simulink model "CartesianSpace_Task"  (R2020b)
settings: Solver=FixedStepDiscrete  StartTime=0.0  StopTime=6  FixedStep=0.01  RelTol=1e-3
undefined symbols (not defined in the file): DiscIntNeverNeededParam
libraries: Utilities x6, robotcorelib x4, simulink x2, XBotBlockToolbox x2

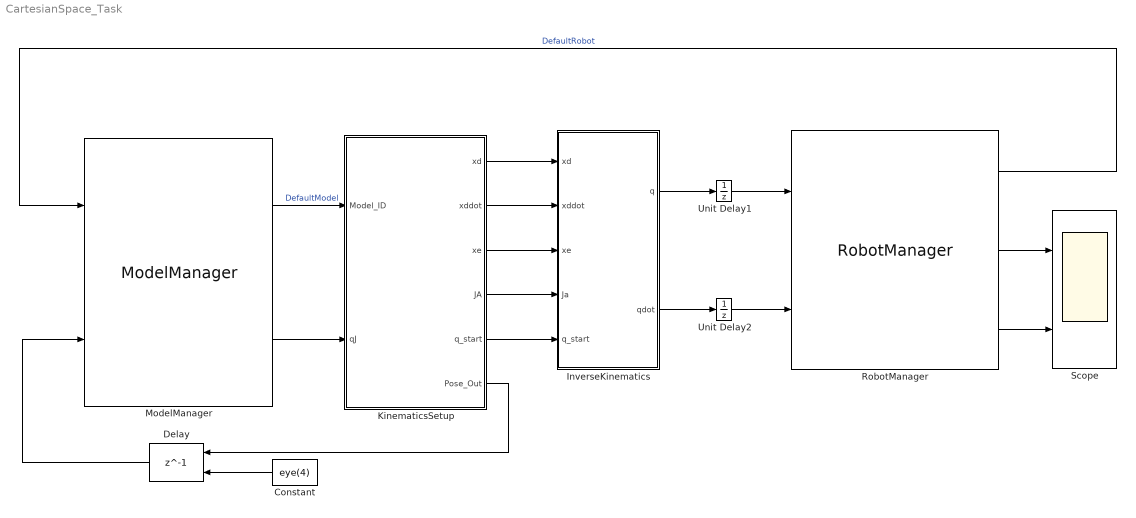
== system CartesianSpace_Task ==
  Constant : Constant  Value=eye(4)
  Delay : Delay  DelayLength=1  InitialConditionSource=Input port  InitialCondition=0
  InverseKinematics : Subsystem
  KinematicsSetup : Subsystem
  ModelManager : XBotBlockToolbox/ModelManager  ModelName=DefaultModel  RobotName=DefaultRobot  UseExtModel=Off  SyncWithRobot=On  GetFloatingBaseList={}  SetFloatingBaseComponent=Pose  GravityRequest=Off  ReadingsList={ 'qJ' }  MechanicalLimitsList={}  MechanicalLimitsCheck=Off  MechanicalLimitsEnforce=Off  SensorList={}  ReferencesList={}  OldModelName=DefaultModel
  RobotManager : XBotBlockToolbox/RobotManager  RobotName=DefaultRobot  ModelName=DefaultModel  UseExtRobot=Off  SyncWithModel=Off  ReadingsList={ 'qJ', 'qJdot' }  MechanicalLimitsList={}  MechanicalLimitsCheck=Off  MechanicalLimitsEnforce=Off  SensorList={}  ReferencesList={ 'qJ_ref', 'qJdot_ref' }  OldRobotName=DefaultRobot
  Scope : Scope  NumInputPorts=2
  Unit Delay1 : UnitDelay  SampleTime=-1  HasFrameUpgradeWarning=on
  Unit Delay2 : UnitDelay  SampleTime=-1  HasFrameUpgradeWarning=on
  wires:
  RobotManager/1 -> ModelManager/1  "DefaultRobot"
  RobotManager/2 -> Scope/1
  RobotManager/3 -> Scope/2
  ModelManager/2 -> KinematicsSetup/2(qJ)
  InverseKinematics/1(q) -> Unit Delay1/1
  InverseKinematics/2(qdot) -> Unit Delay2/1
  ModelManager/1 -> KinematicsSetup/1(Model_ID)  "DefaultModel"
  KinematicsSetup/1(xd) -> InverseKinematics/1(xd)
  KinematicsSetup/2(xddot) -> InverseKinematics/2(xddot)
  KinematicsSetup/3(xe) -> InverseKinematics/3(xe)
  KinematicsSetup/4(JA) -> InverseKinematics/4(Ja)
  Delay/1 -> ModelManager/2
  Constant/1 -> Delay/2
  KinematicsSetup/5(q_start) -> InverseKinematics/5(q_start)
  KinematicsSetup/6(Pose_Out) -> Delay/1
  Unit Delay1/1 -> RobotManager/1
  Unit Delay2/1 -> RobotManager/2

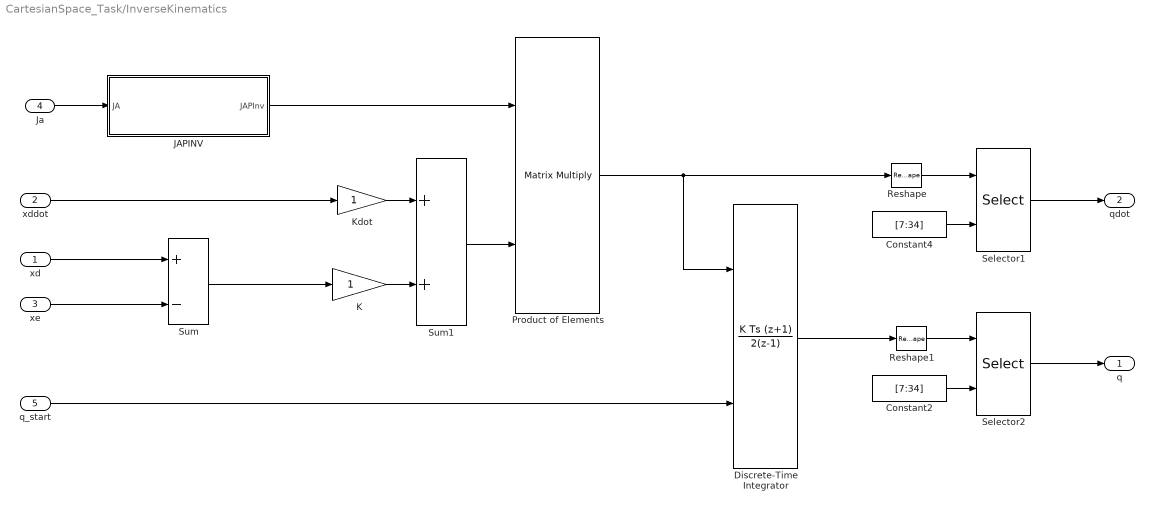
== system CartesianSpace_Task/InverseKinematics ==
  xd : Inport
  xddot : Inport  Port=2
  xe : Inport  Port=3
  Ja : Inport  Port=4
  q_start : Inport  Port=5
  Constant2 : Constant  Value=[7:34]  VectorParams1D=off
  Constant4 : Constant  Value=[7:34]  VectorParams1D=off
  Discrete-Time Integrator : DiscreteIntegrator  IntegratorMethod=Integration: Trapezoidal  InitialConditionSource=external  SampleTime=-1  ICPrevOutput=DiscIntNeverNeededParam  ICPrevScaledInput=DiscIntNeverNeededParam
  JAPINV : MATLAB Function  TreatAsAtomicUnit=on
  K : Gain
  Kdot : Gain
  Product of Elements : Product  Inputs=**  Multiplication=Matrix(*)
  Reshape : Reshape
  Reshape1 : Reshape
  Selector1 : Selector  NumberOfDimensions=2  IndexOptions=Select all,Index vector (port)  Indices=[1 3],1  OutputSizes=1,1
  Selector2 : Selector  NumberOfDimensions=2  IndexOptions=Select all,Index vector (port)  Indices=[1 3],1  OutputSizes=1,1
  Sum : Sum  Inputs=+-
  Sum1 : Sum
  q : Outport
  qdot : Outport  Port=2
  wires:
  xd/1 -> Sum/1
  K/1 -> Sum1/2
  xddot/1 -> Kdot/1
  Kdot/1 -> Sum1/1
  Selector1/1 -> qdot/1
  xe/1 -> Sum/2
  Sum/1 -> K/1
  Sum1/1 -> Product of Elements/2
  JAPINV/1(JAPInv) -> Product of Elements/1
  Ja/1 -> JAPINV/1(JA)
  q_start/1 -> Discrete-Time Integrator/2
  Reshape1/1 -> Selector2/1
  Constant4/1 -> Selector1/2
  Reshape/1 -> Selector1/1
  Discrete-Time Integrator/1 -> Reshape1/1
  Selector2/1 -> q/1
  Constant2/1 -> Selector2/2
  Product of Elements/1 -> Discrete-Time Integrator/1, Reshape/1

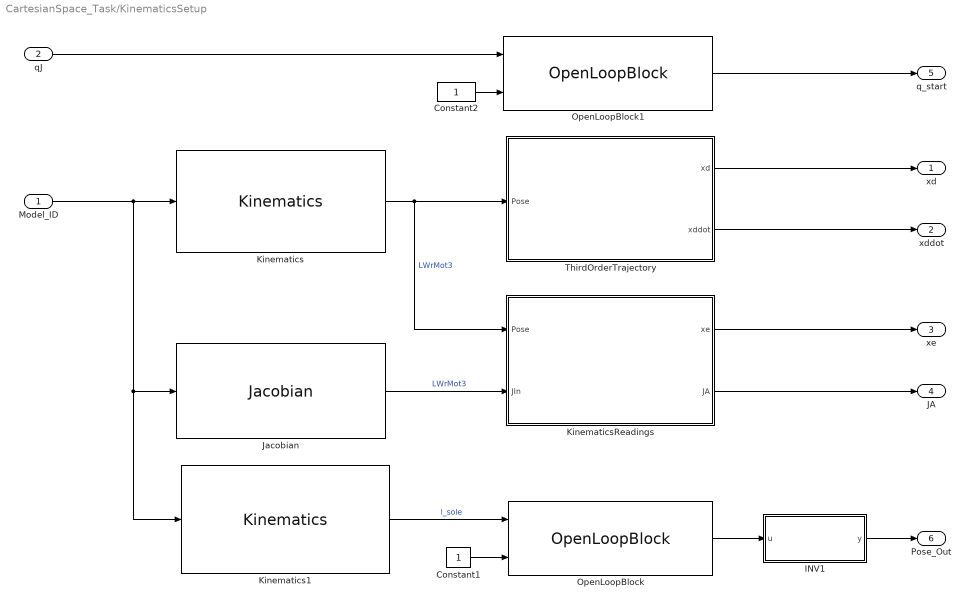
== system CartesianSpace_Task/KinematicsSetup ==
  Model_ID : Inport
  qJ : Inport  Port=2
  Constant1 : Constant
  Constant2 : Constant
  INV1 : MATLAB Function  TreatAsAtomicUnit=on
  Jacobian : Utilities/Jacobian  ModelName=DefaultModel  JacobianList={ 'J' }  LinkName=LWrMot3  ExternalRef=Off
  Kinematics : Utilities/Kinematics  ModelName=DefaultModel  PoseList={ 'Pose' }  SourceFrame=LWrMot3  TwistList={}  COMList={}
  Kinematics1 : Utilities/Kinematics  ModelName=DefaultModel  PoseList={ 'Pose' }  SourceFrame=l_sole  TwistList={}  COMList={}
  KinematicsReadings : Subsystem
  OpenLoopBlock : Utilities/OpenLoopBlock  SystemSampleTime=-1  VariantActivationTime=update diagram  Latency=0  AutoFrameSizeCalculation=off
  OpenLoopBlock1 : Utilities/OpenLoopBlock  SystemSampleTime=-1  VariantActivationTime=update diagram  Latency=0  AutoFrameSizeCalculation=off
  ThirdOrderTrajectory : Subsystem
  xd : Outport
  xddot : Outport  Port=2
  xe : Outport  Port=3
  JA : Outport  Port=4
  q_start : Outport  Port=5
  Pose_Out : Outport  Port=6
  wires:
  Kinematics/1 -> KinematicsReadings/1(Pose), ThirdOrderTrajectory/1(Pose)  "LWrMot3"
  KinematicsReadings/1(xe) -> xe/1
  KinematicsReadings/2(JA) -> JA/1
  Jacobian/1 -> KinematicsReadings/2(JIn)  "LWrMot3"
  Model_ID/1 -> Kinematics/1, Kinematics1/1, Jacobian/1
  ThirdOrderTrajectory/1(xd) -> xd/1
  ThirdOrderTrajectory/2(xddot) -> xddot/1
  OpenLoopBlock/1 -> INV1/1(u)
  INV1/1(y) -> Pose_Out/1
  Kinematics1/1 -> OpenLoopBlock/1  "l_sole"
  Constant1/1 -> OpenLoopBlock/2
  qJ/1 -> OpenLoopBlock1/1
  Constant2/1 -> OpenLoopBlock1/2
  OpenLoopBlock1/1 -> q_start/1

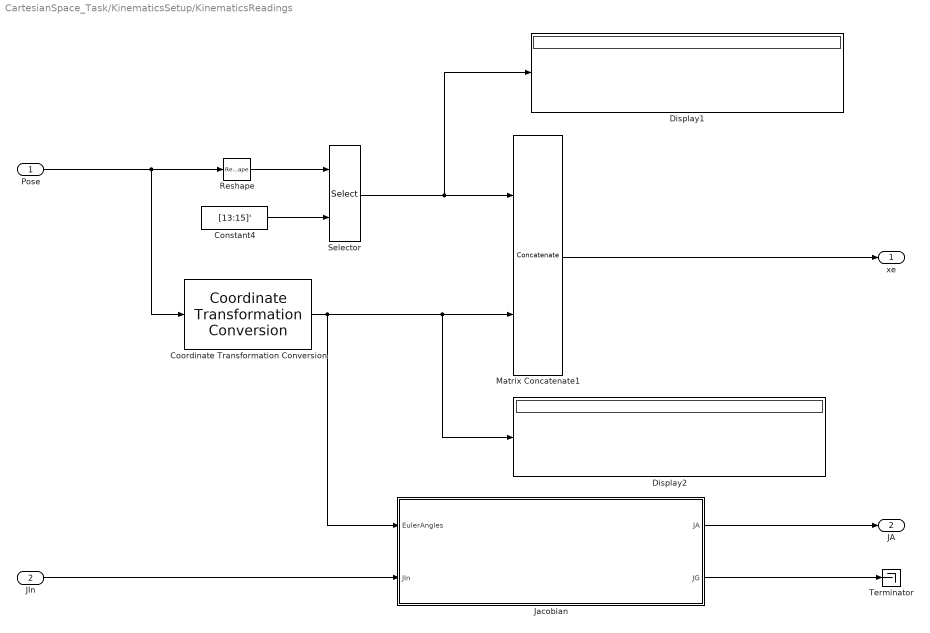
== system CartesianSpace_Task/KinematicsSetup/KinematicsReadings ==
  Pose : Inport
  JIn : Inport  Port=2
  Constant4 : Constant  Value=[13:15]'  VectorParams1D=off
  Coordinate Transformation Conversion : robotcorelib/Coordinate Transformation Conversion  InputRepresentation=Homogeneous Transformation  InputEulerSequence=ZYX  ShowTrVecInputPort=on  OutputRepresentation=Euler Angles  OutputEulerSequence=ZYZ  ShowTrVecOutputPort=off  SimulateUsing=Interpreted execution
  Display1 : Display
  Display2 : Display
  Jacobian : Subsystem
  Matrix Concatenate1 : Concatenate  Mode=Multidimensional array
  Reshape : Reshape  OutputDimensionality=Column vector (2-D)
  Selector : Selector  InputPortWidth=16  IndexOptions=Index vector (port)  Indices=[1 3]  OutputSizes=1
  Terminator : Terminator
  xe : Outport
  JA : Outport  Port=2
  wires:
  Reshape/1 -> Selector/1
  Constant4/1 -> Selector/2
  Matrix Concatenate1/1 -> xe/1
  Jacobian/2(JG) -> Terminator/1
  Jacobian/1(JA) -> JA/1
  Coordinate Transformation Conversion/1 -> Jacobian/1(EulerAngles), Display2/1, Matrix Concatenate1/2
  Selector/1 -> Display1/1, Matrix Concatenate1/1
  Pose/1 -> Coordinate Transformation Conversion/1, Reshape/1
  JIn/1 -> Jacobian/2(JIn)

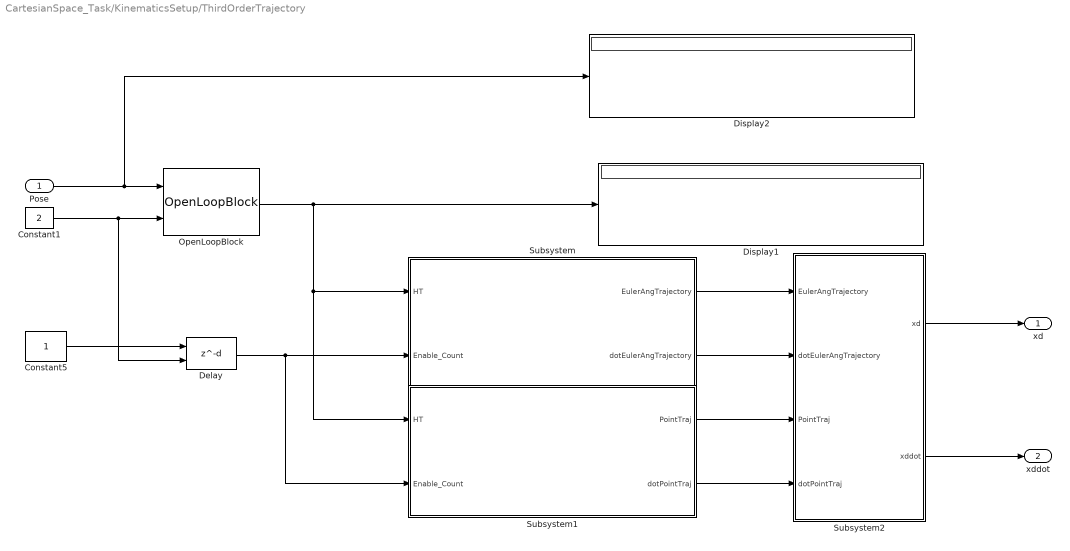
== system CartesianSpace_Task/KinematicsSetup/ThirdOrderTrajectory ==
  Pose : Inport
  Constant1 : Constant  Value=2
  Constant5 : Constant
  Delay : Delay  DelayLengthSource=Input port  DelayLength=1  DelayLengthUpperLimit=600  InitialCondition=0
  Display1 : Display
  Display2 : Display
  OpenLoopBlock : Utilities/OpenLoopBlock  SystemSampleTime=-1  VariantActivationTime=update diagram  Latency=0  AutoFrameSizeCalculation=off
  Subsystem : Subsystem
  Subsystem1 : Subsystem
  Subsystem2 : Subsystem
  xd : Outport
  xddot : Outport  Port=2
  wires:
  Pose/1 -> OpenLoopBlock/1, Display2/1
  Subsystem2/1(xd) -> xd/1
  Subsystem/1(EulerAngTrajectory) -> Subsystem2/1(EulerAngTrajectory)
  Subsystem/2(dotEulerAngTrajectory) -> Subsystem2/2(dotEulerAngTrajectory)
  Subsystem1/1(PointTraj) -> Subsystem2/3(PointTraj)
  Subsystem1/2(dotPointTraj) -> Subsystem2/4(dotPointTraj)
  Subsystem2/2(xddot) -> xddot/1
  Constant5/1 -> Delay/1
  Delay/1 -> Subsystem1/2(Enable_Count), Subsystem/2(Enable_Count)
  OpenLoopBlock/1 -> Subsystem/1(HT), Subsystem1/1(HT), Display1/1
  Constant1/1 -> Delay/2, OpenLoopBlock/2

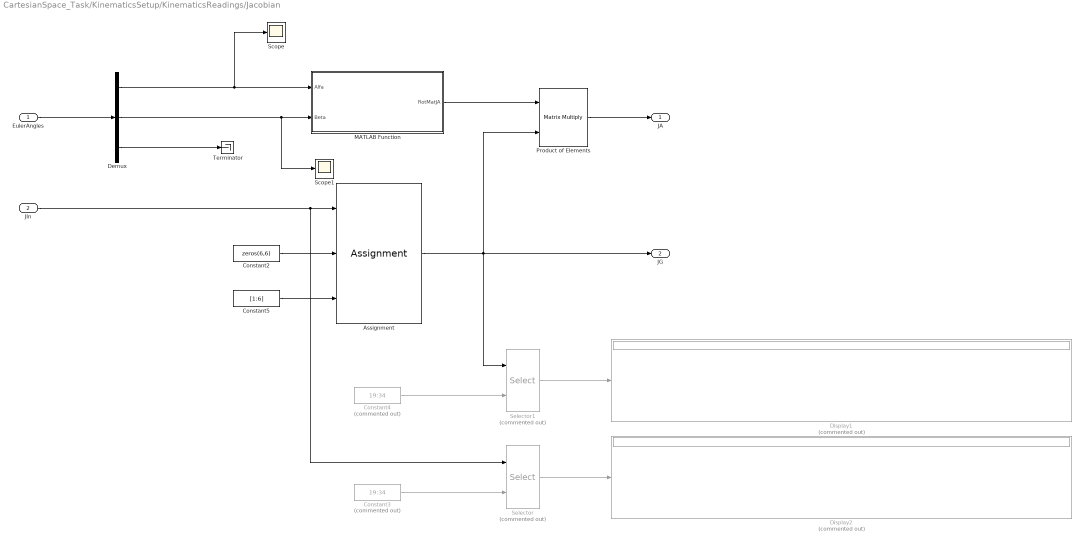
== system CartesianSpace_Task/KinematicsSetup/KinematicsReadings/Jacobian ==
  EulerAngles : Inport
  JIn : Inport  Port=2
  Assignment : Assignment  NumberOfDimensions=2  DiagnosticForDimensions=Warning  IndexOptions=Assign all,Index vector (port)  Indices=1,1  OutputSizes=1,1
  Constant2 : Constant  Value=zeros(6,6)  VectorParams1D=off
  Constant3 : Constant  Commented=on  Value=19:34  VectorParams1D=off
  Constant4 : Constant  Commented=on  Value=19:34  VectorParams1D=off
  Constant5 : Constant  Value=[1:6]  VectorParams1D=off
  Demux : Demux  Outputs=3
  Display1 : Display  Commented=on
  Display2 : Display  Commented=on
  MATLAB Function : MATLAB Function  TreatAsAtomicUnit=on
  Product of Elements : Product  Inputs=**  Multiplication=Matrix(*)
  Scope : Scope
  Scope1 : Scope
  Selector : Selector  Commented=on  NumberOfDimensions=2  IndexOptions=Select all,Index vector (port)  Indices=[1 3],1  OutputSizes=1,1
  Selector1 : Selector  Commented=on  NumberOfDimensions=2  IndexOptions=Select all,Index vector (port)  Indices=[1 3],1  OutputSizes=1,1
  Terminator : Terminator
  JA : Outport
  JG : Outport  Port=2
  wires:
  Constant5/1 -> Assignment/3
  Assignment/1 -> Selector1/1, Product of Elements/2, JG/1
  Constant2/1 -> Assignment/2
  JIn/1 -> Selector/1, Assignment/1
  Demux/1 -> Scope/1, MATLAB Function/1(Alfa)
  Demux/2 -> Scope1/1, MATLAB Function/2(Beta)
  EulerAngles/1 -> Demux/1
  Demux/3 -> Terminator/1
  MATLAB Function/1(RotMatJA) -> Product of Elements/1
  Product of Elements/1 -> JA/1
  Constant3/1 -> Selector/2
  Selector/1 -> Display2/1
  Constant4/1 -> Selector1/2
  Selector1/1 -> Display1/1

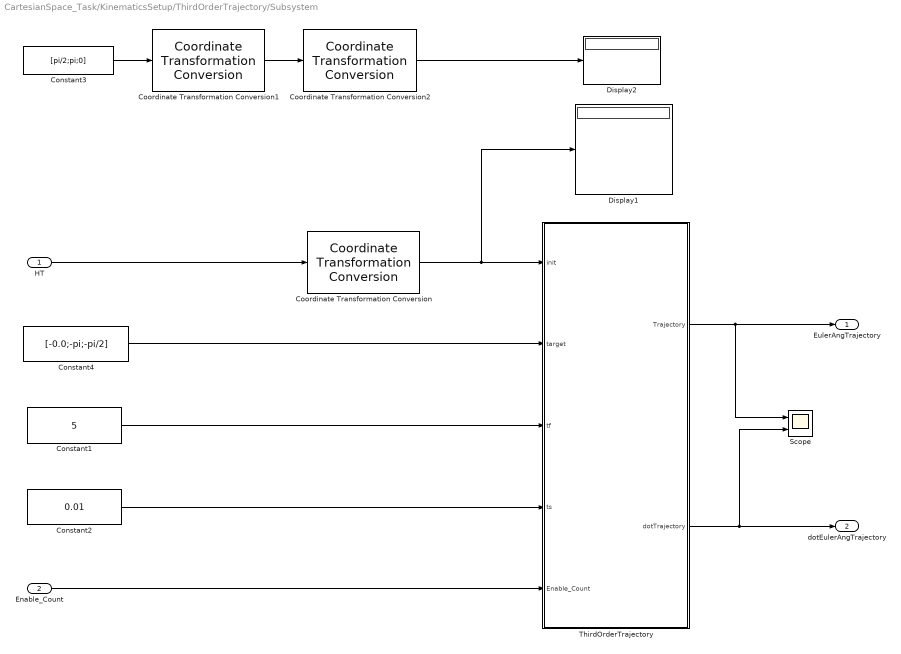
== system CartesianSpace_Task/KinematicsSetup/ThirdOrderTrajectory/Subsystem ==
  HT : Inport
  Enable_Count : Inport  Port=2
  Constant1 : Constant  Value=5
  Constant2 : Constant  Value=0.01
  Constant3 : Constant  Value=[pi/2;pi;0]  VectorParams1D=off
  Constant4 : Constant  Value=[-0.0;-pi;-pi/2]  VectorParams1D=off
  Coordinate Transformation Conversion : robotcorelib/Coordinate Transformation Conversion  InputRepresentation=Homogeneous Transformation  InputEulerSequence=ZYX  ShowTrVecInputPort=on  OutputRepresentation=Euler Angles  OutputEulerSequence=ZYZ  ShowTrVecOutputPort=off  SimulateUsing=Interpreted execution
  Coordinate Transformation Conversion1 : robotcorelib/Coordinate Transformation Conversion  InputRepresentation=Euler Angles  InputEulerSequence=ZYZ  ShowTrVecInputPort=on  OutputRepresentation=Rotation Matrix  OutputEulerSequence=ZYZ  ShowTrVecOutputPort=off  SimulateUsing=Interpreted execution
  Coordinate Transformation Conversion2 : robotcorelib/Coordinate Transformation Conversion  InputRepresentation=Rotation Matrix  InputEulerSequence=ZYX  ShowTrVecInputPort=on  OutputRepresentation=Euler Angles  OutputEulerSequence=ZYZ  ShowTrVecOutputPort=off  SimulateUsing=Interpreted execution
  Display1 : Display
  Display2 : Display
  Scope : Scope  NumInputPorts=2
  ThirdOrderTrajectory : Subsystem
  EulerAngTrajectory : Outport
  dotEulerAngTrajectory : Outport  Port=2
  wires:
  Coordinate Transformation Conversion/1 -> Display1/1, ThirdOrderTrajectory/1(init)
  HT/1 -> Coordinate Transformation Conversion/1
  Constant1/1 -> ThirdOrderTrajectory/3(tf)
  Constant2/1 -> ThirdOrderTrajectory/4(ts)
  ThirdOrderTrajectory/2(dotTrajectory) -> Scope/2, dotEulerAngTrajectory/1
  Enable_Count/1 -> ThirdOrderTrajectory/5(Enable_Count)
  Constant3/1 -> Coordinate Transformation Conversion1/1
  Coordinate Transformation Conversion1/1 -> Coordinate Transformation Conversion2/1
  Coordinate Transformation Conversion2/1 -> Display2/1
  ThirdOrderTrajectory/1(Trajectory) -> EulerAngTrajectory/1, Scope/1
  Constant4/1 -> ThirdOrderTrajectory/2(target)

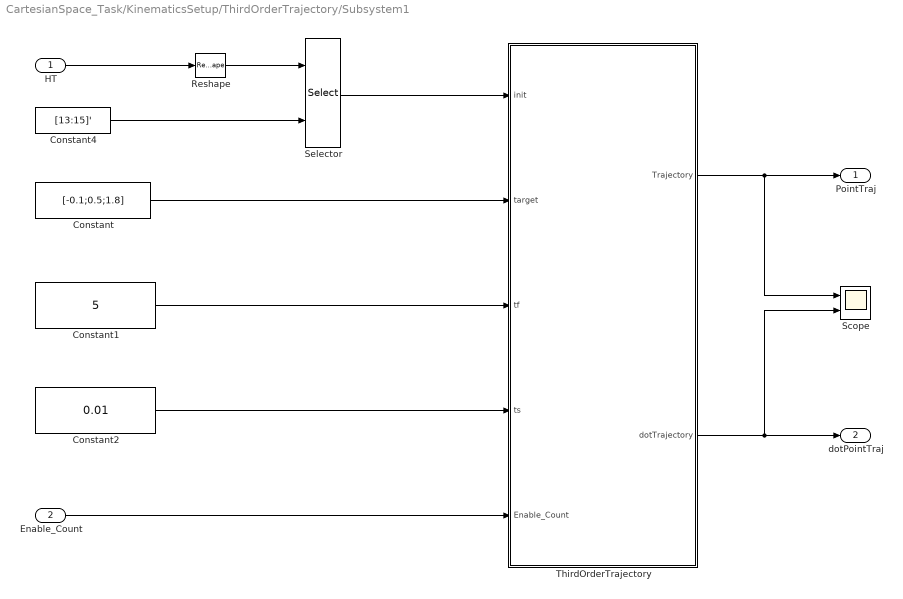
== system CartesianSpace_Task/KinematicsSetup/ThirdOrderTrajectory/Subsystem1 ==
  HT : Inport
  Enable_Count : Inport  Port=2
  Constant : Constant  Value=[-0.1;0.5;1.8]  VectorParams1D=off
  Constant1 : Constant  Value=5
  Constant2 : Constant  Value=0.01
  Constant4 : Constant  Value=[13:15]'  VectorParams1D=off
  Reshape : Reshape  OutputDimensionality=Column vector (2-D)
  Scope : Scope  NumInputPorts=2
  Selector : Selector  InputPortWidth=16  IndexOptions=Index vector (port)  Indices=[1 3]  OutputSizes=1
  ThirdOrderTrajectory : Subsystem
  PointTraj : Outport
  dotPointTraj : Outport  Port=2
  wires:
  Selector/1 -> ThirdOrderTrajectory/1(init)
  ThirdOrderTrajectory/1(Trajectory) -> PointTraj/1, Scope/1
  Constant/1 -> ThirdOrderTrajectory/2(target)
  Constant1/1 -> ThirdOrderTrajectory/3(tf)
  Constant2/1 -> ThirdOrderTrajectory/4(ts)
  Constant4/1 -> Selector/2
  Reshape/1 -> Selector/1
  HT/1 -> Reshape/1
  ThirdOrderTrajectory/2(dotTrajectory) -> Scope/2, dotPointTraj/1
  Enable_Count/1 -> ThirdOrderTrajectory/5(Enable_Count)

== system CartesianSpace_Task/KinematicsSetup/ThirdOrderTrajectory/Subsystem2 ==
  EulerAngTrajectory : Inport
  dotEulerAngTrajectory : Inport  Port=2
  PointTraj : Inport  Port=3
  dotPointTraj : Inport  Port=4
  Matrix Concatenate1 : Concatenate  Mode=Multidimensional array
  Matrix Concatenate2 : Concatenate  Mode=Multidimensional array
  xd : Outport
  xddot : Outport  Port=2
  wires:
  Matrix Concatenate1/1 -> xd/1
  dotPointTraj/1 -> Matrix Concatenate2/1
  EulerAngTrajectory/1 -> Matrix Concatenate1/2
  Matrix Concatenate2/1 -> xddot/1
  dotEulerAngTrajectory/1 -> Matrix Concatenate2/2
  PointTraj/1 -> Matrix Concatenate1/1

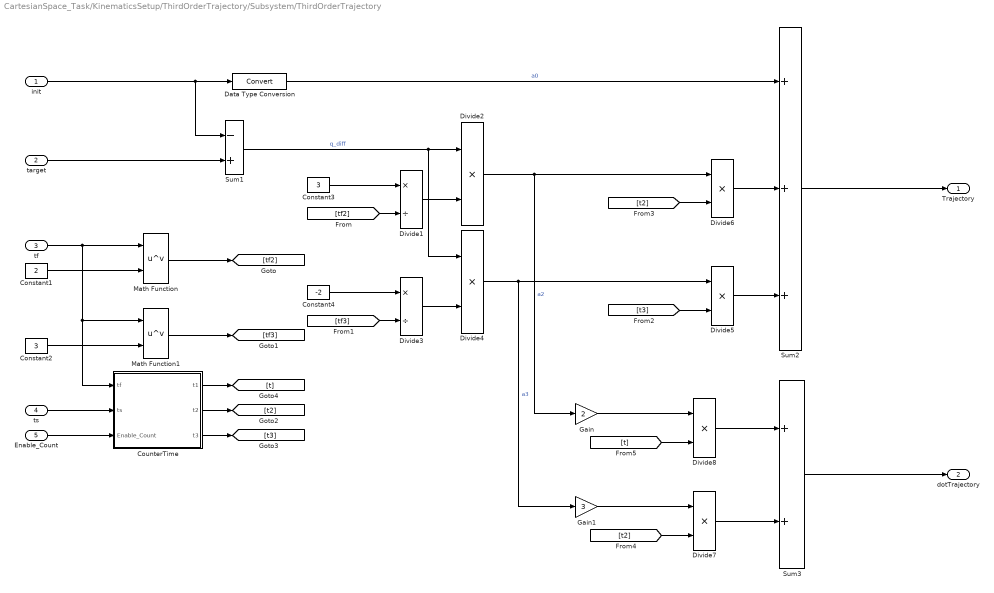
== system CartesianSpace_Task/KinematicsSetup/ThirdOrderTrajectory/Subsystem/ThirdOrderTrajectory ==
  init : Inport
  target : Inport  Port=2
  tf : Inport  Port=3
  ts : Inport  Port=4
  Enable_Count : Inport  Port=5
  Constant1 : Constant  Value=2
  Constant2 : Constant  Value=3
  Constant3 : Constant  Value=3
  Constant4 : Constant  Value=-2
  CounterTime : Subsystem
  Data Type Conversion : DataTypeConversion
  Divide1 : Product  Inputs=*/
  Divide{2,4..8} (6 alike) : Product  Inputs=**
  Divide3 : Product  Inputs=*/
  Gain : Gain  Gain=2
  Gain1 : Gain  Gain=3
  Math Function : Math  Operator=pow  SaturateOnIntegerOverflow=on
  Math Function1 : Math  Operator=pow  SaturateOnIntegerOverflow=on
  Sum1 : Sum  Inputs=-+
  Sum2 : Sum  Inputs=+++
  Sum3 : Sum
  Trajectory : Outport
  dotTrajectory : Outport  Port=2
  wires:
  tf/1 -> CounterTime/1(tf), Math Function1/1, Math Function/1
  Constant1/1 -> Math Function/2
  Constant2/1 -> Math Function1/2
  ts/1 -> CounterTime/2(ts)
  init/1 -> Sum1/1, Data Type Conversion/1
  Sum2/1 -> Trajectory/1
  Math Function1/1 -> [tf3]
  Math Function/1 -> [tf2]
  CounterTime/1(t1) -> [t]
  CounterTime/2(t2) -> [t2]
  CounterTime/3(t3) -> [t3]
  Sum1/1 -> Divide4/1, Divide2/1  "q_diff"
  [tf2] -> Divide1/2
  Constant3/1 -> Divide1/1
  Divide1/1 -> Divide2/2
  Constant4/1 -> Divide3/1
  Divide3/1 -> Divide4/2
  [tf3] -> Divide3/2
  Divide2/1 -> Gain/1, Divide6/1  "a2"
  Divide4/1 -> Gain1/1, Divide5/1  "a3"
  [t3] -> Divide5/2
  [t2] -> Divide6/2
  Data Type Conversion/1 -> Sum2/1  "a0"
  Divide6/1 -> Sum2/2
  Divide5/1 -> Sum2/3
  target/1 -> Sum1/2
  Enable_Count/1 -> CounterTime/3(Enable_Count)
  [t] -> Divide8/2
  Divide8/1 -> Sum3/1
  Divide7/1 -> Sum3/2
  Sum3/1 -> dotTrajectory/1
  [t2] -> Divide7/2
  Gain/1 -> Divide8/1
  Gain1/1 -> Divide7/1

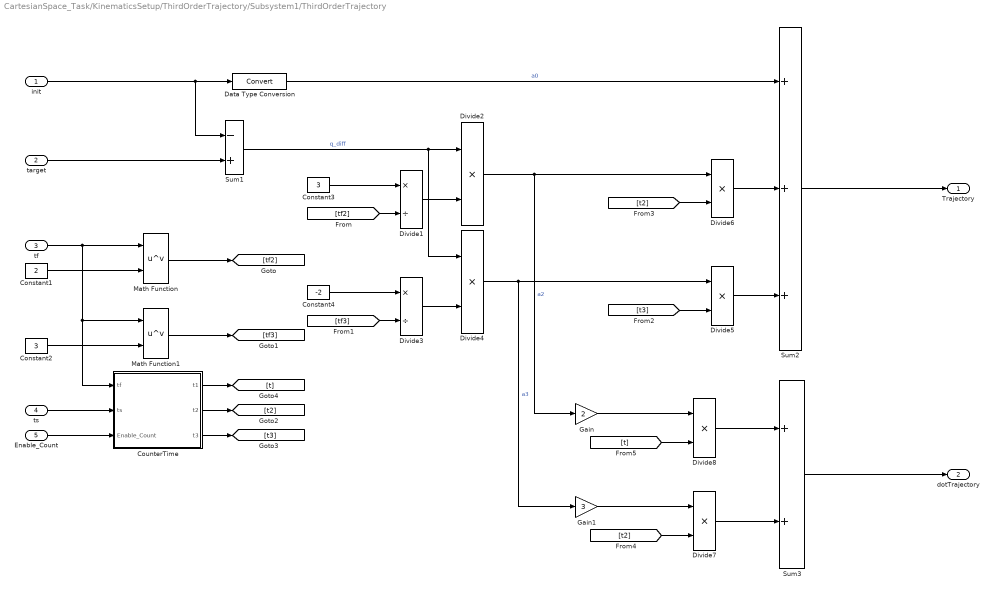
== system CartesianSpace_Task/KinematicsSetup/ThirdOrderTrajectory/Subsystem1/ThirdOrderTrajectory ==
  init : Inport
  target : Inport  Port=2
  tf : Inport  Port=3
  ts : Inport  Port=4
  Enable_Count : Inport  Port=5
  Constant1 : Constant  Value=2
  Constant2 : Constant  Value=3
  Constant3 : Constant  Value=3
  Constant4 : Constant  Value=-2
  CounterTime : Subsystem
  Data Type Conversion : DataTypeConversion
  Divide1 : Product  Inputs=*/
  Divide{2,4..8} (6 alike) : Product  Inputs=**
  Divide3 : Product  Inputs=*/
  Gain : Gain  Gain=2
  Gain1 : Gain  Gain=3
  Math Function : Math  Operator=pow  SaturateOnIntegerOverflow=on
  Math Function1 : Math  Operator=pow  SaturateOnIntegerOverflow=on
  Sum1 : Sum  Inputs=-+
  Sum2 : Sum  Inputs=+++
  Sum3 : Sum
  Trajectory : Outport
  dotTrajectory : Outport  Port=2
  wires:
  tf/1 -> CounterTime/1(tf), Math Function1/1, Math Function/1
  Constant1/1 -> Math Function/2
  Constant2/1 -> Math Function1/2
  ts/1 -> CounterTime/2(ts)
  init/1 -> Sum1/1, Data Type Conversion/1
  Sum2/1 -> Trajectory/1
  Math Function1/1 -> [tf3]
  Math Function/1 -> [tf2]
  CounterTime/1(t1) -> [t]
  CounterTime/2(t2) -> [t2]
  CounterTime/3(t3) -> [t3]
  Sum1/1 -> Divide4/1, Divide2/1  "q_diff"
  [tf2] -> Divide1/2
  Constant3/1 -> Divide1/1
  Divide1/1 -> Divide2/2
  Constant4/1 -> Divide3/1
  Divide3/1 -> Divide4/2
  [tf3] -> Divide3/2
  Divide2/1 -> Gain/1, Divide6/1  "a2"
  Divide4/1 -> Gain1/1, Divide5/1  "a3"
  [t3] -> Divide5/2
  [t2] -> Divide6/2
  Data Type Conversion/1 -> Sum2/1  "a0"
  Divide6/1 -> Sum2/2
  Divide5/1 -> Sum2/3
  target/1 -> Sum1/2
  [t] -> Divide8/2
  Divide8/1 -> Sum3/1
  Divide7/1 -> Sum3/2
  Sum3/1 -> dotTrajectory/1
  [t2] -> Divide7/2
  Gain/1 -> Divide8/1
  Gain1/1 -> Divide7/1
  Enable_Count/1 -> CounterTime/3(Enable_Count)

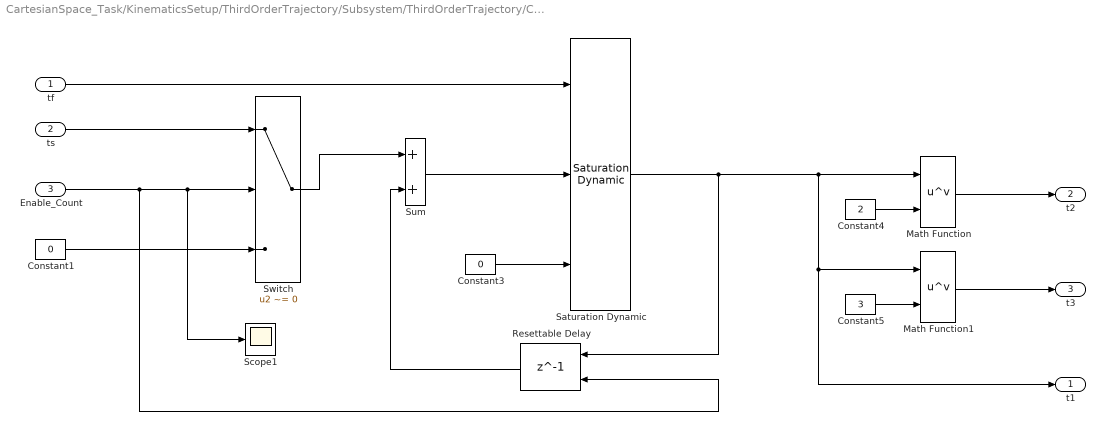
== system CartesianSpace_Task/KinematicsSetup/ThirdOrderTrajectory/Subsystem/ThirdOrderTrajectory/CounterTime ==
  tf : Inport
  ts : Inport  Port=2
  Enable_Count : Inport  Port=3
  Constant1 : Constant  Value=0
  Constant3 : Constant  Value=0
  Constant4 : Constant  Value=2
  Constant5 : Constant  Value=3
  Math Function : Math  Operator=pow  SaturateOnIntegerOverflow=on
  Math Function1 : Math  Operator=pow  SaturateOnIntegerOverflow=on
  Resettable Delay : Delay  DelayLength=1  ExternalReset=Rising
  Saturation Dynamic : simulink/Discontinuities/Saturation Dynamic  OutMin=[]  OutMax=[]  OutDataTypeStr=Inherit: Same as second input  OutDataType=fixdt(1, 16)  OutScaling=2^-10  DoSatur=off
  Scope1 : Scope
  Sum : Sum
  Switch : Switch  Criteria=u2 ~= 0
  t1 : Outport
  t2 : Outport  Port=2
  t3 : Outport  Port=3
  wires:
  Constant3/1 -> Saturation Dynamic/3
  Saturation Dynamic/1 -> Resettable Delay/1, t1/1, Math Function1/1, Math Function/1
  tf/1 -> Saturation Dynamic/1
  ts/1 -> Switch/1
  Sum/1 -> Saturation Dynamic/2
  Resettable Delay/1 -> Sum/2
  Switch/1 -> Sum/1
  Constant1/1 -> Switch/3
  Constant4/1 -> Math Function/2
  Constant5/1 -> Math Function1/2
  Math Function/1 -> t2/1
  Math Function1/1 -> t3/1
  Enable_Count/1 -> Resettable Delay/2, Scope1/1, Switch/2

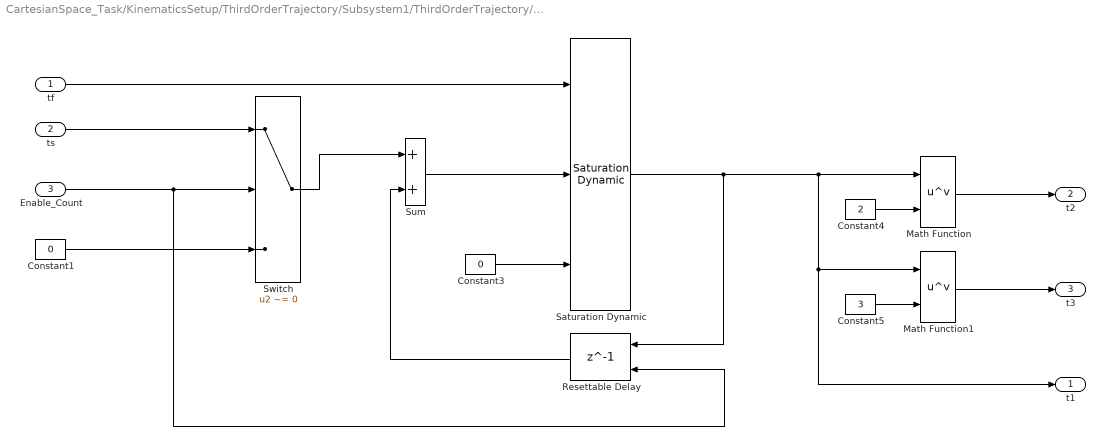
== system CartesianSpace_Task/KinematicsSetup/ThirdOrderTrajectory/Subsystem1/ThirdOrderTrajectory/CounterTime ==
  tf : Inport
  ts : Inport  Port=2
  Enable_Count : Inport  Port=3
  Constant1 : Constant  Value=0
  Constant3 : Constant  Value=0
  Constant4 : Constant  Value=2
  Constant5 : Constant  Value=3
  Math Function : Math  Operator=pow  SaturateOnIntegerOverflow=on
  Math Function1 : Math  Operator=pow  SaturateOnIntegerOverflow=on
  Resettable Delay : Delay  DelayLength=1  ExternalReset=Rising
  Saturation Dynamic : simulink/Discontinuities/Saturation Dynamic  OutMin=[]  OutMax=[]  OutDataTypeStr=Inherit: Same as second input  OutDataType=fixdt(1, 16)  OutScaling=2^-10  DoSatur=off
  Sum : Sum
  Switch : Switch  Criteria=u2 ~= 0
  t1 : Outport
  t2 : Outport  Port=2
  t3 : Outport  Port=3
  wires:
  Constant3/1 -> Saturation Dynamic/3
  Saturation Dynamic/1 -> Resettable Delay/1, t1/1, Math Function1/1, Math Function/1
  tf/1 -> Saturation Dynamic/1
  ts/1 -> Switch/1
  Sum/1 -> Saturation Dynamic/2
  Resettable Delay/1 -> Sum/2
  Switch/1 -> Sum/1
  Constant1/1 -> Switch/3
  Constant4/1 -> Math Function/2
  Constant5/1 -> Math Function1/2
  Math Function/1 -> t2/1
  Math Function1/1 -> t3/1
  Enable_Count/1 -> Resettable Delay/2, Switch/2

== matlab function CartesianSpace_Task/InverseKinematics/JAPINV ==
function JAPInv = pseudoinverse(JA)

JAPInv=pinv(JA);

== matlab function CartesianSpace_Task/KinematicsSetup/INV1 ==
function y = fcn(u)

y = inv(u);

== matlab function CartesianSpace_Task/KinematicsSetup/KinematicsReadings/Jacobian/MATLAB Function ==
function RotMatJA = RotMatrixJAGeneration(Alfa,Beta)

RotMatJA=zeros(6,6);
RotMatJA(1:3,1:3)=eye(3);
RA=[0,-sin(Alfa),cos(Alfa)*sin(Beta);0,cos(Alfa),sin(Alfa)*sin(Beta);1,0,cos(Beta)];
RAi=inv(RA);
RotMatJA(4:6,4:6)=RAi;
